simulink library "libMdl_RecordedData"  (R2019b)
settings: Solver=VariableStepAuto  StartTime=0.0  StopTime=10.0  RelTol=1e-3
undefined symbols (not defined in the file): gnss_sample_time, gnss_sim_data, gnss_sim_data_validity, time_gnss
settings Model: Creator=Hanno  LastModifiedBy=Hanno

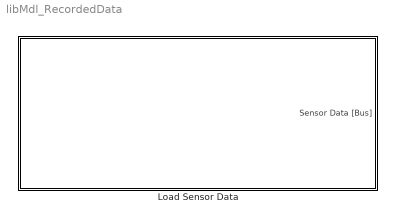
== system libMdl_RecordedData ==
  Load Sensor Data : Subsystem  mask(Load Sensor Data From Workspace){mv_input_data=gnss_sim_data, mv_data_validity=gnss_sim_data_validity, mv_input_time=time_gnss, mv_sample_time=gnss_sample_time}
      mask prompts: mv_input_data "Input Data:"; mv_data_validity "Validity Data:"; mv_input_time "Input Time:"; mv_sample_time "Sample Time:"
      mask help:
      | Loads sensor data from workspace, i.e. data which has a data sequence together with a corresponding time vetor.
      |
      | Each simulink time step the data is output by utilizing zero order hold interpolation. Additionally, a valid bit is appended at the end of the signal. It is only true, when the simulink time matches a multiple of the specified sample time of this block.
      |
      | Input Data: Data in timeseries format (consider data organization: row wise or column wise in the further processing steps)
      |
      | Validity Data: Data validity flag as timeseries.
      |
      | Input Time: Sensor specific time relative to the simulink simulation time.
      |
      | Sample Time: Sampling rate of the sensor data. Each time the simulink time matches a multiple of the sample time the data is marked as valid.
      mask Display:
      | str1 = sprintf('\\color{black}{\\bfRecorded Sensor Data}\n\n');
      | str2 = sprintf('Sample Time: %0.3f\n\n',mv_sample_time);
      | 
      | str = [str1,str2];
      | 
      | text( 0.5,0.5, ...
      |       str, ...
      |       'horizontalAlignment', 'center', ...
      |       'texmode','on' ...
      |     )

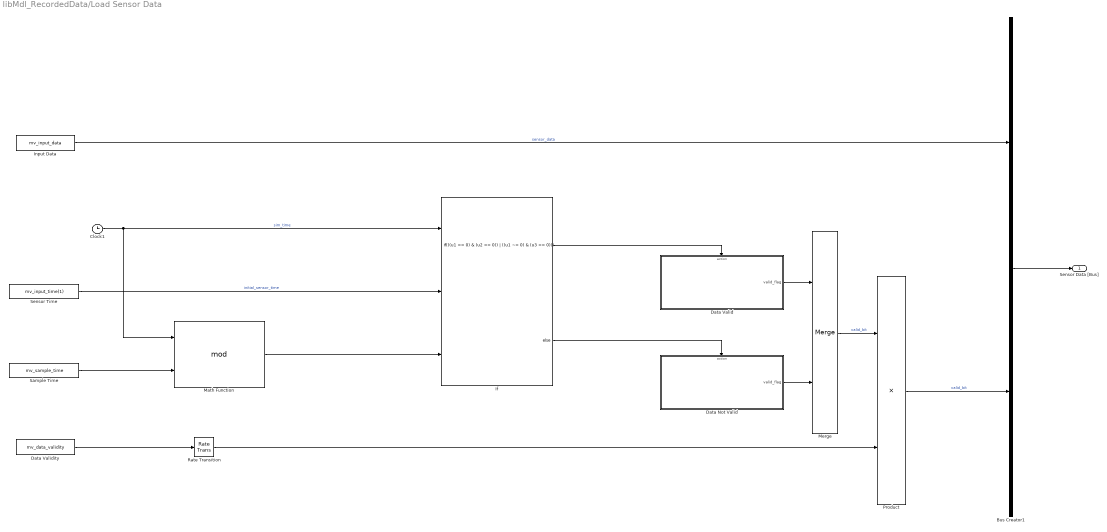
== system libMdl_RecordedData/Load Sensor Data ==
  Bus Creator1 : BusCreator  Inputs=2
  Clock1 : Clock
  Data Not Valid : Subsystem  TreatAsAtomicUnit=on
  Data Valid : Subsystem  TreatAsAtomicUnit=on
  Data Validity : FromWorkspace  VariableName=mv_data_validity  SampleTime=0  Interpolate=off  OutputAfterFinalValue=Holding final value
  If : If  NumInputs=3  IfExpression=((u1 == 0) & (u2 == 0)) | ((u1 ~= 0) & (u3 == 0))
  Input Data : FromWorkspace  VariableName=mv_input_data  SampleTime=mv_sample_time  Interpolate=off  OutputAfterFinalValue=Setting to zero
  Math Function : Math  Operator=mod  SignedPower=off  SaturateOnIntegerOverflow=on
  Merge : Merge
  Product : Product
  Rate Transition : RateTransition  InitialCondition=mv_data_validity.Data(1)
  Sample Time : Constant  Value=mv_sample_time
  Sensor Time : Constant  Value=mv_input_time(1)
  Sensor Data [Bus] : Outport
  wires:
  Rate Transition/1 -> Product/2
  Math Function/1 -> If/3
  Input Data/1 -> Bus Creator1/1  "sensor_data"
  Sample Time/1 -> Math Function/2
  Clock1/1 -> Math Function/1, If/1  "sim_time"
  Data Valid/1(valid_flag) -> Merge/1
  Sensor Time/1 -> If/2  "initial_sensor_time"
  Product/1 -> Bus Creator1/2  "valid_bit"
  Bus Creator1/1 -> Sensor Data [Bus]/1
  Data Not Valid/1(valid_flag) -> Merge/2
  If/1 -> Data Valid/Action
  If/2 -> Data Not Valid/Action
  Merge/1 -> Product/1  "valid_bit"
  Data Validity/1 -> Rate Transition/1

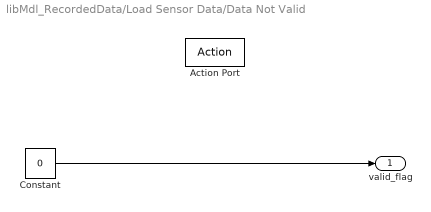
== system libMdl_RecordedData/Load Sensor Data/Data Not Valid ==
  Action Port : ActionPort
  Constant : Constant  Value=0
  valid_flag : Outport
  wires:
  Constant/1 -> valid_flag/1

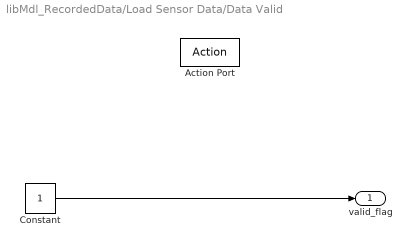
== system libMdl_RecordedData/Load Sensor Data/Data Valid ==
  Action Port : ActionPort
  Constant : Constant
  valid_flag : Outport
  wires:
  Constant/1 -> valid_flag/1
